simulink model "digital_communication_network"  (R2022b)
settings: Solver=VariableStepAuto  StartTime=0.0  StopTime=T  MaxStep=MaxStep  RelTol=RelTol
undefined symbols (not defined in the file): J, T, X0
libraries: HyEQ_Library x2
settings Model: Creator=tom  LastModifiedBy=tom

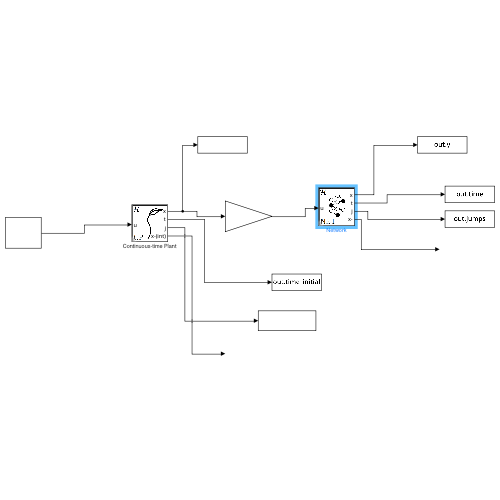
[thumbnail: Simulink's stored preview of the top-level diagram]
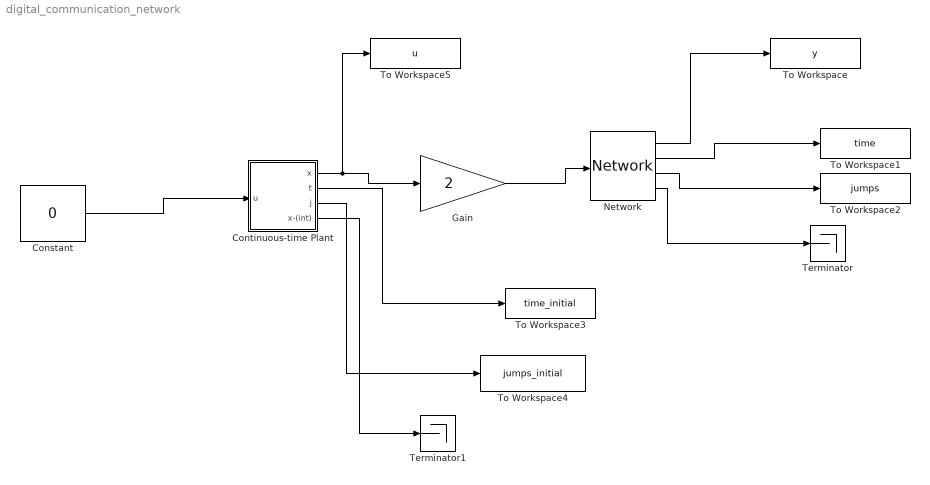
== system digital_communication_network ==
  Constant : Constant  Value=0
  Continuous-time Plant : Subsystem  LoadFcn=set_param(gcb,'LinkStatus','none')  mask(Continuous Process){z0=X0, input_dim=1, parameters=[], T=T}
      mask prompts: z0 "Initial State (column vector)"; input_dim "Input dimension (nonnegative integer)"; T "Flow Horizon (nonnegative real)"
      mask help:
      | To define the continuous process:
      | 1. Select the block,
      | 2. "Look inside" the block: Either open the context menu and select Mask > Look Under Mask, or click the arrow in the bottom-left corner of the block.
      | 3. Edit the "flow map f" block to define the continuous dynamics.
      | 4. Edit the "flow set C" block to define the region where the continuous process is allowed to flow.
      mask init:
      | state_dim = size(z0, 1);
      settings: CopyFcn=|
      | set_param(gcb,'LinkStatus','none'),
      | set_param(gcs, 'MaxStep', 'MaxStep', 'RelTol', 'RelTol','StopTime', 'T')
      mask Help: eval hybrid.internal.openHelp('Example_vehicle_on_path')
      mask TypeOptions T: Integrator System/T
      mask DialogControl Control2 Prompt: CPS Components Documentation
      mask DialogControl Control2 Callback: hybrid.internal.openHelp('CPS_Components')
      mask DialogControl ParameterGroupVar Prompt: Configuration
      mask Display:
      | image('Cplant.jpg')
      | port_label('output', 1, 'x')
      | port_label('output', 2, 't')
      | port_label('output', 3, 'j')
      | port_label('output', 4, 'x-(int)')
      | port_label('input', 1, 'u')
  Gain : Gain  Gain=2
  Network : HyEQ_Library/Cyber Physical Systems/Network  T_min=T_min  T_max=T_max  ms_0=y0  tau_0=tau_0  T=T  J=J
      settings: SourceProductName=Hybrid Equations Toolbox
  Terminator : Terminator
  Terminator1 : Terminator
  To Workspace : ToWorkspace  VariableName=y  SaveFormat=Timeseries  SampleTime=-1
  To Workspace1 : ToWorkspace  VariableName=time  SaveFormat=Timeseries  SampleTime=-1
  To Workspace2 : ToWorkspace  VariableName=jumps  SaveFormat=Timeseries  SampleTime=-1
  To Workspace3 : ToWorkspace  VariableName=time_initial  SaveFormat=Timeseries  SampleTime=-1
  To Workspace4 : ToWorkspace  VariableName=jumps_initial  SaveFormat=Timeseries  SampleTime=-1
  To Workspace5 : ToWorkspace  VariableName=u  SaveFormat=Timeseries  SampleTime=-1
  wires:
  Constant/1 -> Continuous-time Plant/1(u)
  Continuous-time Plant/1(x) -> To Workspace5/1, Gain/1
  Gain/1 -> Network/1
  Network/1 -> To Workspace/1
  Network/4 -> Terminator/1
  Network/3 -> To Workspace2/1
  Network/2 -> To Workspace1/1
  Continuous-time Plant/4(x-(int)) -> Terminator1/1
  Continuous-time Plant/2(t) -> To Workspace3/1
  Continuous-time Plant/3(j) -> To Workspace4/1

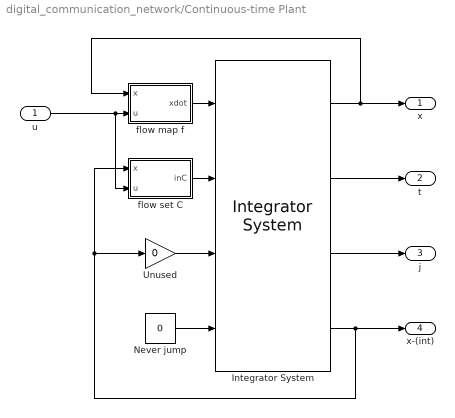
== system digital_communication_network/Continuous-time Plant ==
  u : Inport  PortDimensions=input_dim
  Integrator System : HyEQ_Library/Other/Integrator System  Priority=2  T=T  J=1  x0=z0  rule=1
      settings: SourceProductName=Hybrid Equations Toolbox
  Never jump : Constant  Value=0
  Unused : Gain  Gain=0
  flow map f : MATLAB Function  TreatAsAtomicUnit=on
  flow set C : MATLAB Function  TreatAsAtomicUnit=on
  x : Outport  PortDimensions=state_dim
  t : Outport  Port=2  PortDimensions=1
  j : Outport  Port=3  PortDimensions=1
  x-(int) : Outport  Port=4  PortDimensions=state_dim
  wires:
  Unused/1 -> Integrator System/3
  Never jump/1 -> Integrator System/4
  u/1 -> flow map f/2(u), flow set C/2(u)
  Integrator System/3 -> j/1
  Integrator System/2 -> t/1
  flow set C/1(inC) -> Integrator System/2
  Integrator System/1 -> x/1, flow map f/1(x)
  Integrator System/4 -> x-(int)/1, flow set C/1(x), Unused/1
  flow map f/1(xdot) -> Integrator System/1

== matlab function digital_communication_network/Continuous-time Plant/flow map f ==
  data: x input size=state_dim; xdot output size=state_dim; u input size=input_dim
function xdot = f(x, u)
    % Define the flow map for the continuous process here.
    xdot_1 = -x(1) + u;
    xdot_2 = u + 1;
    xdot_3 = u - 2 + x(1);
    xdot = [xdot_1;xdot_2;xdot_3];
end

== matlab function digital_communication_network/Continuous-time Plant/flow set C ==
  data: x input size=state_dim; inC output size=1; u input size=input_dim
function inC = C(x, u)
    % Define the flow set indicator function for the continuous process here.
    inC = 1;
end
